simulink model "ReducedDynamicsVOR"  (R2025a)
settings: Solver=ode45  StartTime=0.0  StopTime=2000  RelTol=1e-3
values from neighbouring files (symbols this model uses):
  SS_red = ss(A_red, B_red, C_red, D_red)    [FindF16Dynamics_VOR.m]
undefined symbols (not defined in the file or in its folder): trim_state_lo
libraries: simulink_extras x2, slpidlib x1
settings Model: Creator=rohitroychowdhury  LastModifiedBy=rohitroychowdhury

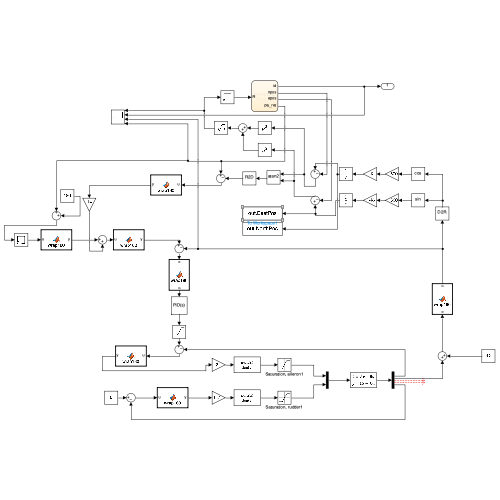
[thumbnail: Simulink's stored preview of the top-level diagram]
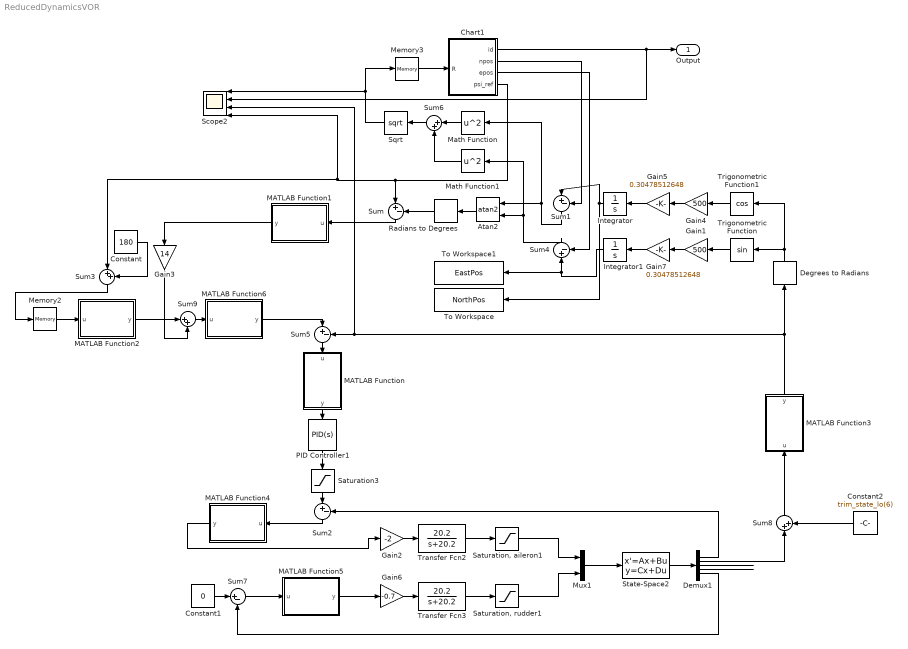
== system ReducedDynamicsVOR ==
  Atan2 : Trigonometry  Operator=atan2
  Chart1 : Stateflow chart  TreatAsAtomicUnit=on
  Constant : Constant  Value=180
  Constant1 : Constant  Value=0
  Constant2 : Constant  Value=trim_state_lo(6)
  Degrees to Radians : simulink_extras/Transformations/Degrees to Radians
  Demux1 : Demux  Outputs=5
  Gain1 : Gain  Gain=500
  Gain2 : Gain  Gain=-2
  Gain3 : Gain  Gain=14
  Gain4 : Gain  Gain=500
  Gain5 : Gain  Gain=0.30478512648
  Gain6 : Gain  Gain=-0.7
  Gain7 : Gain  Gain=0.30478512648
  Integrator : Integrator
  Integrator1 : Integrator
  MATLAB Function : MATLAB Function  TreatAsAtomicUnit=on
  MATLAB Function1 : MATLAB Function  TreatAsAtomicUnit=on
  MATLAB Function2 : MATLAB Function  TreatAsAtomicUnit=on
  MATLAB Function3 : MATLAB Function  TreatAsAtomicUnit=on
  MATLAB Function4 : MATLAB Function  TreatAsAtomicUnit=on
  MATLAB Function5 : MATLAB Function  TreatAsAtomicUnit=on
  MATLAB Function6 : MATLAB Function  TreatAsAtomicUnit=on
  Math Function : Math  Operator=square
  Math Function1 : Math  Operator=square
  Memory2 : Memory
  Memory3 : Memory
  Mux1 : Mux  Inputs=2
  PID Controller1 : slpidlib/PID Controller  Controller=PID  Form=Parallel  TimeDomain=Continuous-time  UseExternalTs=off  SampleTime=-1  IntegratorMethod=Forward Euler  FilterMethod=Forward Euler  ControllerParametersSource=internal  P=10  I=0.01  UseKiTs=off  D=30  UseExternalDerivativeSource=off  N=100  UseFilter=on  TunerSelectOption=Transfer Function Based (PID Tuner App)  InitialConditionSource=internal  InitialConditionForIntegrator=0  InitialConditionForFilter=0  DifferentiatorICPrevScaledInput=0  ExternalReset=none  TrackingMode=off  Kt=1  LimitOutput=off  SatLimitsSource=internal  UpperSaturationLimit=inf  LowerSaturationLimit=-inf  LinearizeAsGain=on  AntiWindupMode=none  Kb=1  LimitIntegrator=off  UpperIntegratorSaturationLimit=inf  LowerIntegratorSaturationLimit=-inf  POutMin=[]  POutMax=[]  IOutMin=[]  IOutMax=[]  DOutMin=[]  DOutMax=[]  NOutMin=[]  NOutMax=[]  SumOutMin=[]  SumOutMax=[]  SaturationOutMin=[]  SaturationOutMax=[]  PParamMin=[]  PParamMax=[]  IParamMin=[]  IParamMax=[]  DParamMin=[]  DParamMax=[]  NParamMin=[]  NParamMax=[]  KbParamMin=[]  KbParamMax=[]  KtParamMin=[]  KtParamMax=[]  KbOutMin=[]  KbOutMax=[]  KtOutMin=[]  KtOutMax=[]  IntegratorOutMin=[]  IntegratorOutMax=[]  FilterOutMin=[]  FilterOutMax=[]  SumI1OutMin=[]  SumI1OutMax=[]  SumI2OutMin=[]  SumI2OutMax=[]  SumI3OutMin=[]  SumI3OutMax=[]  SumI4OutMin=[]  SumI4OutMax=[]  SumDOutMin=[]  SumDOutMax=[]  DifferentiatorOutMin=[]  DifferentiatorOutMax=[]  FilterDiffOutCoefMin=[]  FilterDiffOutCoefMax=[]  ReciprocalOutMin=[]  ReciprocalOutMax=[]  SumDenOutMin=[]  SumDenOutMax=[]  SumNumOutMin=[]  SumNumOutMax=[]  DivideOutMin=[]  DivideOutMax=[]  UdiffTsProdOutMin=[]  UdiffTsProdOutMax=[]  NTsProdOutMin=[]  NTsProdOutMax=[]  UintegralTsProdOutMin=[]  UintegralTsProdOutMax=[]  UngainTsProdOutMin=[]  UngainTsProdOutMax=[]  ClampingZeroOutDataTypeStr=Inherit: Inherit via back propagation  ClampingZeroOutMin=[]  ClampingZeroOutMax=[]  FilterDenConstantOutDataTypeStr=Inherit: Inherit via back propagation  FilterDenConstantOutMin=[]  FilterDenConstantOutMax=[]  PCopyOutDataTypeStr=Inherit: Inherit via back propagation  PCopyOutMin=[]  PCopyOutMax=[]  NCopyOutDataTypeStr=Inherit: Inherit via back propagation  NCopyOutMin=[]  NCopyOutMax=[]  IntegratorContinuousStateAttributes=''  IntegratorStateMustResolveToSignalObject=off  IntegratorRTWStateStorageClass=Auto  FilterContinuousStateAttributes=''  FilterStateMustResolveToSignalObject=off  FilterRTWStateStorageClass=Auto  ParallelPVariant=InternalParameters  IdealPVariant=Disabled  IVariant=InternalParameters  DVariant=InternalParameters  IntegratorVariant=Continuous  SatVariant=Disabled  AWVariant=Passthrough  PCopyVariant=Disabled  TRVariant=Disabled  FdbkBlocksVariant=Forward  IdealPFdbkVariant=Disabled  SatFdbkVariant=Disabled  DerivativeFilterVariant=ContFilter  NVariant=InternalParameters  NCopyVariant=Disabled  FilterICVariant=InternalICsFilter  IntegratorICVariant=InternalICs  ExternalResetVariant=Disabled  TRSumVariant=Passthrough  SumFdbkVariant=Disabled  SumVariant=Sum_PID  TsampFilterVariant=InternalTs  TsampNgainVariant=Passthrough  TsampIntegralVariant=Disabled_SignalSpec  ExternalSaturationOutDataTypeStr=Inherit: Same as second input  DerivativeSourceVariant=ErrorSignal  PreIntVariant=InternalPreInt
  Radians to Degrees : simulink_extras/Transformations/Radians to Degrees
  "Saturation, aileron1" : Saturate  UpperLimit=21.5  LowerLimit=-21.5
  "Saturation, rudder1" : Saturate  UpperLimit=30  LowerLimit=-30
  Saturation3 : Saturate  UpperLimit=45  LowerLimit=-45
  Scope2 : Scope  NumInputPorts=4
      settings: ActiveDisplayYMinimum=-796.5620258832887  ActiveDisplayYMaximum=57022.929253668291  DataLoggingVariableName=ScopeData2
  Sqrt : Sqrt
  State-Space2 : StateSpace  A=SS_red.A  B=SS_red.B  C=SS_red.C  D=SS_red.D  InitialCondition=0
  Sum{,1..2,4..5,7} (6 alike) : Sum  Inputs=|+-
  Sum{3,6,8..9} (4 alike) : Sum  Inputs=|++
  To Workspace : ToWorkspace  VariableName=NorthPos  SaveFormat=Timeseries  SampleTime=-1
  To Workspace1 : ToWorkspace  VariableName=EastPos  SaveFormat=Timeseries  SampleTime=-1
  Transfer Fcn2 : TransferFcn  Numerator=[20.2]  Denominator=[1 20.2]
  Transfer Fcn3 : TransferFcn  Numerator=[20.2]  Denominator=[1 20.2]
  Trigonometric Function : Trigonometry  ApproximationMethod=CORDIC
  Trigonometric Function1 : Trigonometry  Operator=cos  ApproximationMethod=CORDIC
  Output : Outport
  wires:
  Demux1/3 -> ?
  Mux1/1 -> State-Space2/1
  Saturation3/1 -> Sum2/1
  Gain2/1 -> Transfer Fcn2/1
  MATLAB Function/1(y) -> PID Controller1/1
  Sum2/1 -> MATLAB Function4/1(u)
  Demux1/1 -> Sum2/2
  "Saturation, rudder1"/1 -> Mux1/2
  Demux1/4 -> ?
  "Saturation, aileron1"/1 -> Mux1/1
  Transfer Fcn2/1 -> "Saturation, aileron1"/1
  Transfer Fcn3/1 -> "Saturation, rudder1"/1
  State-Space2/1 -> Demux1/1
  Degrees to Radians/1 -> Trigonometric Function1/1, Trigonometric Function/1
  Trigonometric Function1/1 -> Gain4/1
  Trigonometric Function/1 -> Gain1/1
  Gain1/1 -> Gain7/1
  Gain4/1 -> Gain5/1
  Sum4/1 -> Atan2/2, Math Function1/1
  Sum1/1 -> Atan2/1, Math Function/1
  Chart1/1(id) -> Scope2/2, Output/1
  Math Function/1 -> Sum6/1
  Math Function1/1 -> Sum6/2
  Sum6/1 -> Sqrt/1
  Sqrt/1 -> Memory3/1, Scope2/1
  Memory3/1 -> Chart1/1(R)
  Gain7/1 -> Integrator1/1
  Gain5/1 -> Integrator/1
  Demux1/5 -> Sum7/2
  Sum7/1 -> MATLAB Function5/1(u)
  Gain6/1 -> Transfer Fcn3/1
  Constant1/1 -> Sum7/1
  Integrator1/1 -> To Workspace1/1, Sum4/1
  Chart1/3(epos) -> Sum4/2
  Integrator/1 -> To Workspace/1, Sum1/1
  Chart1/2(npos) -> Sum1/2
  Constant2/1 -> Sum8/2
  Demux1/2 -> Sum8/1
  Chart1/4(psi_ref) -> Sum/1, Sum3/1, Scope2/4
  Atan2/1 -> Radians to Degrees/1
  Radians to Degrees/1 -> Sum/2
  Sum/1 -> MATLAB Function1/1(u)
  Sum5/1 -> MATLAB Function/1(u)
  MATLAB Function1/1(y) -> Gain3/1
  Constant/1 -> Sum3/2
  Sum3/1 -> Memory2/1
  Sum9/1 -> MATLAB Function6/1(u)
  Sum8/1 -> MATLAB Function3/1(u)
  MATLAB Function4/1(y) -> Gain2/1
  MATLAB Function5/1(y) -> Gain6/1
  Gain3/1 -> Sum9/2
  MATLAB Function2/1(y) -> Sum9/1
  Memory2/1 -> MATLAB Function2/1(u)
  PID Controller1/1 -> Saturation3/1
  MATLAB Function3/1(y) -> Scope2/3, Sum5/2, Degrees to Radians/1
  MATLAB Function6/1(y) -> Sum5/1

== matlab function ReducedDynamicsVOR/MATLAB Function1 ==
  data: u input; y output
function y = wrap180(u)
% Wrap angle to [-180, 180)

y = mod(u + 180, 360) - 180;

== matlab function ReducedDynamicsVOR/MATLAB Function ==
  data: u input; y output
function y = wrap180(u)
% Wrap angle to [-180, 180)

y = mod(u + 180, 360) - 180;

== stateflow chart ReducedDynamicsVOR/Chart1 ==
  settings: updateMethod=DISCRETE  sampleTime=0.1
  state beacon1
    id=1;
    npos=15000;
    epos=15000;
    psi_ref=45;
  state beacon2
    id=2;
    npos=0;
    epos=30000;
    psi_ref=135;
  state beacon3
    id=3;
    npos=-15000;
    epos=30000;
    psi_ref=180;
  state beacon4
    id=4;
    npos=-30000;
    epos=45000;
    psi_ref=135;
  state beacon5
    id=5;
    npos=0;
    epos=0;
    psi_ref=0;
  (default) -> beacon1
  beacon2 -> beacon3 : [R<5000]
  beacon3 -> beacon4 : [R<5000]
  beacon1 -> beacon2 : [R<5000]
  beacon4 -> beacon5 : [R<5000]
  beacon5 -> beacon1 : [R<5000]
  data: R input; id output; npos output; epos output; psi_ref output

== matlab function ReducedDynamicsVOR/MATLAB Function2 ==
  data: u input; y output
function y = wrap180(u)
% Wrap angle to [-180, 180)

y = mod(u + 180, 360) - 180;

== matlab function ReducedDynamicsVOR/MATLAB Function3 ==
  data: u input; y output
function y = wrap180(u)
% Wrap angle to [-180, 180)

y = mod(u + 180, 360) - 180;

== matlab function ReducedDynamicsVOR/MATLAB Function4 ==
  data: u input; y output
function y = wrap180(u)
% Wrap angle to [-180, 180)

y = mod(u + 180, 360) - 180;

== matlab function ReducedDynamicsVOR/MATLAB Function5 ==
  data: u input; y output
function y = wrap180(u)
% Wrap angle to [-180, 180)

y = mod(u + 180, 360) - 180;

== matlab function ReducedDynamicsVOR/MATLAB Function6 ==
  data: u input; y output
function y = wrap180(u)
% Wrap angle to [-180, 180)

y = mod(u + 180, 360) - 180;
